simulink model "model2v6"  (R2020b)
settings: Solver=VariableStepAuto  StartTime=0.0  StopTime=10.0  RelTol=1e-3
settings Model: Creator=dkravchenko  LastModifiedBy=dkravchenko

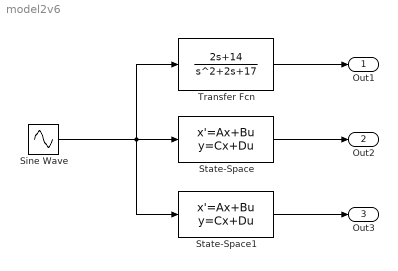
== system model2v6 ==
  Sine Wave : Sin  Amplitude=0  Bias=1  Frequency=0  SampleTime=0
  State-Space : StateSpace  A=[0 1; -17 -2]  B=[0; 1]  C=[14 2]  D=0  InitialCondition=0
  State-Space1 : StateSpace  A=[0 -17; 1 -2]  B=[14; 2]  C=[0 1]  D=0  InitialCondition=0
  Transfer Fcn : TransferFcn  Numerator=[2 14]  Denominator=[1 2 17]
  Out1 : Outport
  Out2 : Outport  Port=2
  Out3 : Outport  Port=3
  wires:
  State-Space1/1 -> Out3/1
  Sine Wave/1 -> State-Space1/1, Transfer Fcn/1, State-Space/1
  Transfer Fcn/1 -> Out1/1
  State-Space/1 -> Out2/1
